simulink model "Q_estimation"  (R2021a)
settings: Solver=ode3  StartTime=0.0  StopTime=40  FixedStep=t_sim  RelTol=1e-3
values from neighbouring files (symbols this model uses):
  B0 = [0.1331 -0.0121 0.3981]    [Q_parameter.m]
  eul_0 = [0;0;0]    [Q_parameter.m]    (also in R_parameter.m)
  G0 = [0 0 9.81]    [Q_parameter.m]    (also in R_parameter.m = [0; 0; 9.81])
  k = 1    [Q_parameter.m]
  la = 9e-2    (= 0.09)    [Q_parameter.m]
  lc = 5e-2    (= 0.05)    [Q_parameter.m]
  ma = 9e-3    (= 0.009)    [Q_parameter.m]
  mc = 5e-3    (= 0.005)    [Q_parameter.m]
undefined symbols (not defined in the file or in its folder): DiscIntNeverNeededParam
libraries: sharedtransform x6, aerolibutil x4, sharedutil x3
settings Model: Creator=quangtruc  LastModifiedBy=quangtruc

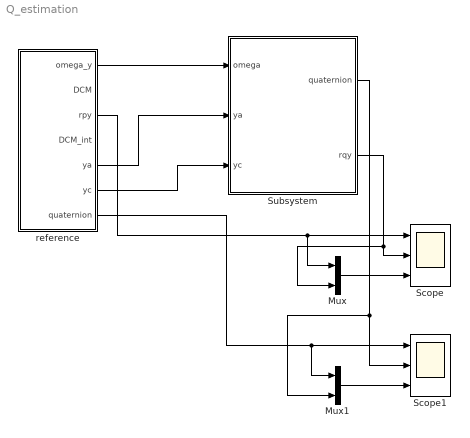
== system Q_estimation ==
  Mux : Mux  Inputs=2
  Mux1 : Mux  Inputs=2
  Scope : Scope  NumInputPorts=3
  Scope1 : Scope  NumInputPorts=3
  Subsystem : Subsystem
  reference : Subsystem
  wires:
  reference/1(omega_y) -> Subsystem/1(omega)
  reference/5(ya) -> Subsystem/2(ya)
  reference/6(yc) -> Subsystem/3(yc)
  Mux1/1 -> Scope1/3
  Mux/1 -> Scope/3
  Subsystem/2(rqy) -> Mux/2, Scope/2
  reference/3(rpy) -> Mux/1, Scope/1
  Subsystem/1(quaternion) -> Mux1/2, Scope1/2
  reference/7(quaternion) -> Scope1/1, Mux1/1

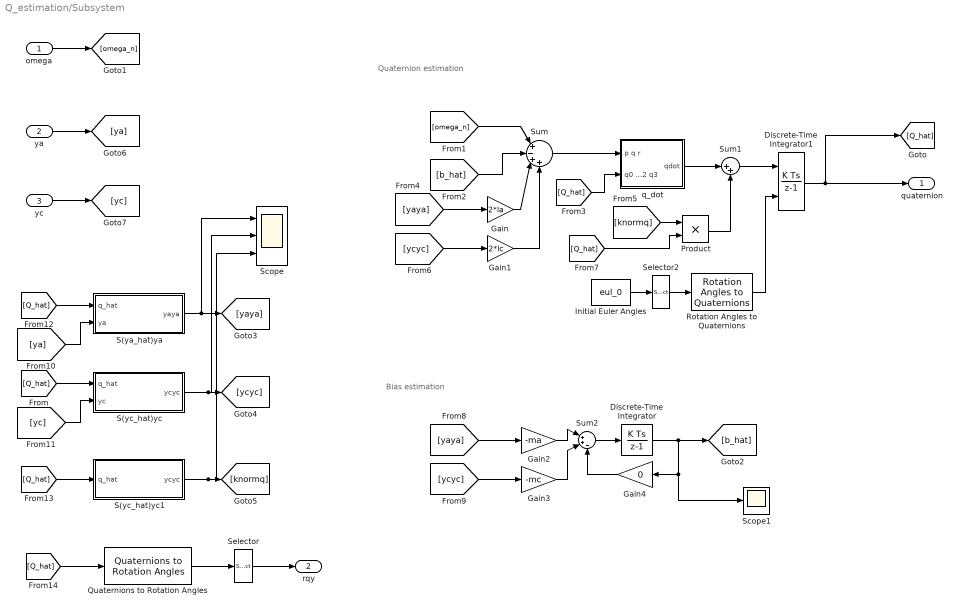
== system Q_estimation/Subsystem ==
  note: Bias estimation
  note: Quaternion estimation
  omega : Inport
  ya : Inport  Port=2
  yc : Inport  Port=3
  Discrete-Time Integrator : DiscreteIntegrator  SampleTime=-1  ICPrevOutput=DiscIntNeverNeededParam  ICPrevScaledInput=DiscIntNeverNeededParam
  Discrete-Time Integrator1 : DiscreteIntegrator  InitialConditionSource=external  SampleTime=-1  ICPrevOutput=DiscIntNeverNeededParam  ICPrevScaledInput=DiscIntNeverNeededParam
  Gain : Gain  Gain=2*la
  Gain1 : Gain  Gain=2*lc
  Gain2 : Gain  Gain=-ma
  Gain3 : Gain  Gain=-mc
  Gain4 : Gain  Gain=0
  Initial Euler Angles : Constant  Value=eul_0
  Product : Product
  Quaternions to Rotation Angles : sharedtransform/Quaternions to Rotation Angles  rotationOrder=ZYX  aMode=aMode
      settings: SourceProductBaseCode=AE,PW,DR,MT,UV,VE
  Rotation Angles to Quaternions : sharedtransform/Rotation Angles to Quaternions  rotationOrder=ZYX  aMode=aMode
      settings: SourceProductBaseCode=AE,PW,DR,MT,UV,VE
  S(ya_hat)ya : Subsystem
  S(yc_hat)yc : Subsystem
  S(yc_hat)yc1 : Subsystem
  Scope : Scope  NumInputPorts=3
  Scope1 : Scope
  Selector : Selector  InputPortWidth=3  IndexOptions=Index vector (dialog)  Indices=[3 2 1]  OutputSizes=1
  Selector2 : Selector  InputPortWidth=3  IndexOptions=Index vector (dialog)  Indices=[3 2 1]  OutputSizes=1
  Sum : Sum  Inputs=|+-++
  Sum1 : Sum  Inputs=|++
  Sum2 : Sum  Inputs=|++-
  q_dot : Subsystem
  quaternion : Outport  VectorParamsAs1DForOutWhenUnconnected=off
  rqy : Outport  Port=2  VectorParamsAs1DForOutWhenUnconnected=off
  wires:
  Initial Euler Angles/1 -> Selector2/1
  Rotation Angles to Quaternions/1 -> Discrete-Time Integrator1/2
  Discrete-Time Integrator1/1 -> [Q_hat], quaternion/1
  Selector2/1 -> Rotation Angles to Quaternions/1
  [omega_n] -> Sum/1
  Sum/1 -> q_dot/1(p q r)
  [b_hat] -> Sum/2
  Sum1/1 -> Discrete-Time Integrator1/1
  [Q_hat] -> q_dot/2(q0 q1 q2 q3)
  [yaya] -> Gain/1
  [ycyc] -> Gain1/1
  Gain/1 -> Sum/3
  Gain1/1 -> Sum/4
  [knormq] -> Product/1
  [Q_hat] -> Product/2
  [ycyc] -> Gain3/1
  [yaya] -> Gain2/1
  Gain2/1 -> Sum2/1
  Gain3/1 -> Sum2/2
  Sum2/1 -> Discrete-Time Integrator/1
  Discrete-Time Integrator/1 -> Gain4/1, Scope1/1, [b_hat]
  omega/1 -> [omega_n]
  ya/1 -> [ya]
  yc/1 -> [yc]
  [Q_hat] -> S(ya_hat)ya/1(q_hat)
  S(ya_hat)ya/1(yaya) -> Scope/1, [yaya]
  S(yc_hat)yc/1(ycyc) -> Scope/2, [ycyc]
  [Q_hat] -> S(yc_hat)yc/1(q_hat)
  [ya] -> S(ya_hat)ya/2(ya)
  [yc] -> S(yc_hat)yc/2(yc)
  S(yc_hat)yc1/1(ycyc) -> Scope/3, [knormq]
  [Q_hat] -> S(yc_hat)yc1/1(q_hat)
  Quaternions to Rotation Angles/1 -> Selector/1
  [Q_hat] -> Quaternions to Rotation Angles/1
  Selector/1 -> rqy/1
  Gain4/1 -> Sum2/3
  q_dot/1(qdot) -> Sum1/1
  Product/1 -> Sum1/2

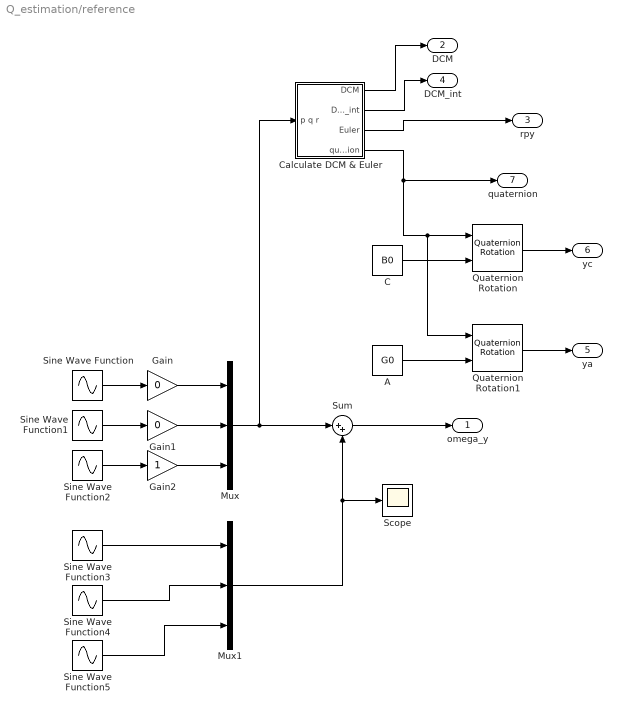
== system Q_estimation/reference ==
  A : Constant  Value=G0
  C : Constant  Value=B0
  "Calculate DCM & Euler " : Subsystem
  Gain : Gain  Gain=0
  Gain1 : Gain  Gain=0
  Gain2 : Gain
  Mux : Mux  Inputs=3
  Mux1 : Mux  Inputs=3
  Quaternion Rotation : aerolibutil/Quaternion Rotation
  Quaternion Rotation1 : aerolibutil/Quaternion Rotation
  Scope : Scope
  Sine Wave Function : Sin  SampleTime=0
  Sine Wave Function1 : Sin  SampleTime=0
  Sine Wave Function2 : Sin  Amplitude=0.5  Frequency=0.5  SampleTime=0
  Sine Wave Function3 : Sin  Amplitude=0.01  Frequency=0.1  SampleTime=0
  Sine Wave Function4 : Sin  Amplitude=0.015  Frequency=0.02  SampleTime=0
  Sine Wave Function5 : Sin  Amplitude=0.011  Frequency=0.005  SampleTime=0
  Sum : Sum  Inputs=|++
  omega_y : Outport
  DCM : Outport  Port=2
  rpy : Outport  Port=3
  DCM_int : Outport  Port=4
  ya : Outport  Port=5
  yc : Outport  Port=6
  quaternion : Outport  Port=7
  wires:
  "Calculate DCM & Euler "/1(DCM) -> DCM/1
  "Calculate DCM & Euler "/2(DCM_int) -> DCM_int/1
  "Calculate DCM & Euler "/3(Euler) -> rpy/1
  Gain/1 -> Mux/1
  Sine Wave Function/1 -> Gain/1
  Sine Wave Function1/1 -> Gain1/1
  Sine Wave Function2/1 -> Gain2/1
  Gain1/1 -> Mux/2
  Gain2/1 -> Mux/3
  Mux/1 -> "Calculate DCM & Euler "/1("p q r "), Sum/1
  Mux1/1 -> Scope/1, Sum/2
  Sum/1 -> omega_y/1
  "Calculate DCM & Euler "/4(quaternion) -> quaternion/1, Quaternion Rotation1/1, Quaternion Rotation/1
  C/1 -> Quaternion Rotation/2
  Quaternion Rotation/1 -> yc/1
  A/1 -> Quaternion Rotation1/2
  Quaternion Rotation1/1 -> ya/1
  Sine Wave Function3/1 -> Mux1/1
  Sine Wave Function4/1 -> Mux1/2
  Sine Wave Function5/1 -> Mux1/3

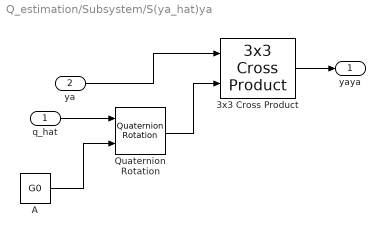
== system Q_estimation/Subsystem/S(ya_hat)ya ==
  q_hat : Inport
  ya : Inport  Port=2
  3x3 Cross Product : sharedutil/3x3 Cross Product  aMode=aMode
      settings: SourceProductBaseCode=AE,PW,DR,MT,UV,VE
  A : Constant  Value=G0
  Quaternion Rotation : aerolibutil/Quaternion Rotation
  yaya : Outport
  wires:
  q_hat/1 -> Quaternion Rotation/1
  A/1 -> Quaternion Rotation/2
  3x3 Cross Product/1 -> yaya/1
  ya/1 -> 3x3 Cross Product/1
  Quaternion Rotation/1 -> 3x3 Cross Product/2

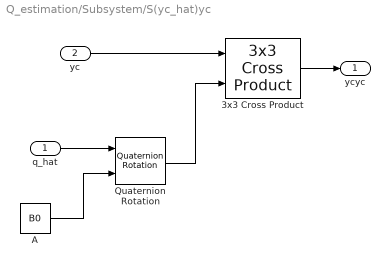
== system Q_estimation/Subsystem/S(yc_hat)yc ==
  q_hat : Inport
  yc : Inport  Port=2
  3x3 Cross Product : sharedutil/3x3 Cross Product  aMode=aMode
      settings: SourceProductBaseCode=AE,PW,DR,MT,UV,VE
  A : Constant  Value=B0
  Quaternion Rotation : aerolibutil/Quaternion Rotation
  ycyc : Outport
  wires:
  q_hat/1 -> Quaternion Rotation/1
  A/1 -> Quaternion Rotation/2
  3x3 Cross Product/1 -> ycyc/1
  yc/1 -> 3x3 Cross Product/1
  Quaternion Rotation/1 -> 3x3 Cross Product/2

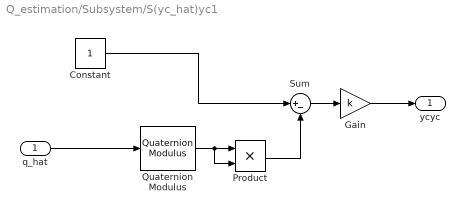
== system Q_estimation/Subsystem/S(yc_hat)yc1 ==
  q_hat : Inport
  Constant : Constant
  Gain : Gain  Gain=k
  Product : Product
  Quaternion Modulus : sharedutil/Quaternion Modulus  aMode=aMode
      settings: SourceProductBaseCode=AE,PW,DR,MT,UV,VE
  Sum : Sum  Inputs=|+-
  ycyc : Outport
  wires:
  Gain/1 -> ycyc/1
  q_hat/1 -> Quaternion Modulus/1
  Quaternion Modulus/1 -> Product/2, Product/1
  Product/1 -> Sum/2
  Sum/1 -> Gain/1
  Constant/1 -> Sum/1

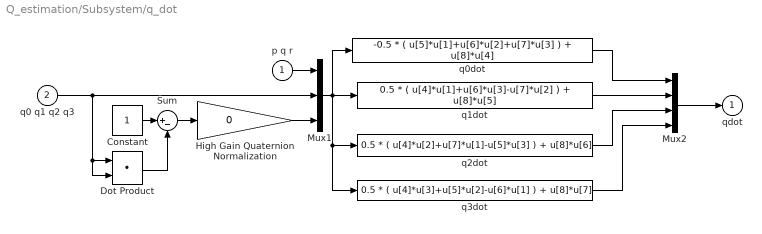
== system Q_estimation/Subsystem/q_dot ==
  p q r : Inport
  q0 q1 q2 q3 : Inport  Port=2
  Constant : Constant
  Dot Product : DotProduct  OutDataTypeStr=Inherit: Inherit via internal rule
  High Gain Quaternion Normalization : Gain  Gain=0  SaturateOnIntegerOverflow=on  OutDataTypeStr=Inherit: Same as input  ParamDataTypeStr=Inherit: Same as input
  Mux1 : Mux  Inputs=[3 4 1]
  Mux2 : Mux
  Sum : Sum  Inputs=|+-  InputSameDT=on  SaturateOnIntegerOverflow=on  OutDataTypeStr=Inherit: Same as first input
  q0dot : Fcn  Expr=-0.5 * ( u[5]*u[1]+u[6]*u[2]+u[7]*u[3] ) + u[8]*u[4]
  q1dot : Fcn  Expr=0.5 * ( u[4]*u[1]+u[6]*u[3]-u[7]*u[2] ) + u[8]*u[5]
  q2dot : Fcn  Expr=0.5 * ( u[4]*u[2]+u[7]*u[1]-u[5]*u[3] ) + u[8]*u[6]
  q3dot : Fcn  Expr=0.5 * ( u[4]*u[3]+u[5]*u[2]-u[6]*u[1] ) + u[8]*u[7]
  qdot : Outport  InitialOutput=0  VectorParamsAs1DForOutWhenUnconnected=off
  wires:
  q0 q1 q2 q3/1 -> Dot Product/1, Dot Product/2, Mux1/2
  q0dot/1 -> Mux2/1
  Constant/1 -> Sum/1
  Mux1/1 -> q2dot/1, q3dot/1, q0dot/1, q1dot/1
  Mux2/1 -> qdot/1
  q2dot/1 -> Mux2/3
  p q r/1 -> Mux1/1
  High Gain Quaternion Normalization/1 -> Mux1/3
  Dot Product/1 -> Sum/2
  q3dot/1 -> Mux2/4
  Sum/1 -> High Gain Quaternion Normalization/1
  q1dot/1 -> Mux2/2

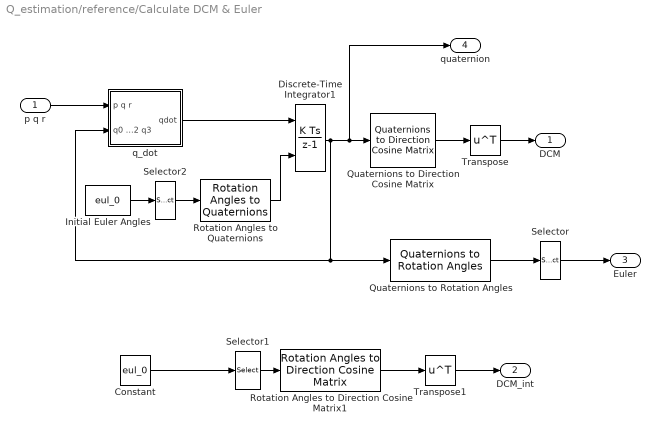
== system Q_estimation/reference/Calculate DCM & Euler  ==
  "p q r " : Inport
  Constant : Constant  Value=eul_0
  Discrete-Time Integrator1 : DiscreteIntegrator  InitialConditionSource=external  SampleTime=-1  ICPrevOutput=DiscIntNeverNeededParam  ICPrevScaledInput=DiscIntNeverNeededParam
  Initial Euler Angles : Constant  Value=eul_0
  Quaternions to Direction Cosine Matrix : sharedtransform/Quaternions to  Direction Cosine Matrix  aMode=aMode
      settings: SourceProductBaseCode=AE,PW,DR,MT,UV,VE
  Quaternions to Rotation Angles : sharedtransform/Quaternions to Rotation Angles  rotationOrder=ZYX  aMode=aMode
      settings: SourceProductBaseCode=AE,PW,DR,MT,UV,VE
  Rotation Angles to Direction Cosine Matrix1 : sharedtransform/Rotation Angles to Direction Cosine Matrix  rotationOrder=ZYX  aMode=aMode
      settings: SourceProductBaseCode=AE,PW,DR,MT,UV,VE
  Rotation Angles to Quaternions : sharedtransform/Rotation Angles to Quaternions  rotationOrder=ZYX  aMode=aMode
      settings: SourceProductBaseCode=AE,PW,DR,MT,UV,VE
  Selector : Selector  InputPortWidth=3  IndexOptions=Index vector (dialog)  Indices=[3 2 1]  OutputSizes=1
  Selector1 : Selector  InputPortWidth=3  IndexOptions=Index vector (dialog)  Indices=[3 2 1]  OutputSizes=1
  Selector2 : Selector  InputPortWidth=3  IndexOptions=Index vector (dialog)  Indices=[3 2 1]  OutputSizes=1
  Transpose : Math  Operator=transpose  SignedPower=on  SaturateOnIntegerOverflow=on
  Transpose1 : Math  Operator=transpose  SignedPower=on  SaturateOnIntegerOverflow=on
  q_dot : Subsystem
  DCM : Outport  VectorParamsAs1DForOutWhenUnconnected=off
  DCM_int : Outport  Port=2  VectorParamsAs1DForOutWhenUnconnected=off
  Euler : Outport  Port=3  VectorParamsAs1DForOutWhenUnconnected=off
  quaternion : Outport  Port=4  VectorParamsAs1DForOutWhenUnconnected=off
  wires:
  Rotation Angles to Direction Cosine Matrix1/1 -> Transpose1/1
  Transpose1/1 -> DCM_int/1
  Selector1/1 -> Rotation Angles to Direction Cosine Matrix1/1
  Constant/1 -> Selector1/1
  Quaternions to Rotation Angles/1 -> Selector/1
  "p q r "/1 -> q_dot/1(p q r)
  Initial Euler Angles/1 -> Selector2/1
  q_dot/1(qdot) -> Discrete-Time Integrator1/1
  Rotation Angles to Quaternions/1 -> Discrete-Time Integrator1/2
  Selector2/1 -> Rotation Angles to Quaternions/1
  Discrete-Time Integrator1/1 -> quaternion/1, Quaternions to Direction Cosine Matrix/1, q_dot/2(q0 q1 q2 q3), Quaternions to Rotation Angles/1
  Quaternions to Direction Cosine Matrix/1 -> Transpose/1
  Transpose/1 -> DCM/1
  Selector/1 -> Euler/1

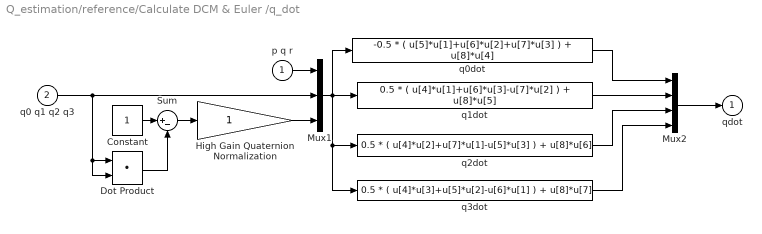
== system Q_estimation/reference/Calculate DCM & Euler /q_dot ==
  p q r : Inport
  q0 q1 q2 q3 : Inport  Port=2
  Constant : Constant
  Dot Product : DotProduct  OutDataTypeStr=Inherit: Inherit via internal rule
  High Gain Quaternion Normalization : Gain  SaturateOnIntegerOverflow=on  OutDataTypeStr=Inherit: Same as input  ParamDataTypeStr=Inherit: Same as input
  Mux1 : Mux  Inputs=[3 4 1]
  Mux2 : Mux
  Sum : Sum  Inputs=|+-  InputSameDT=on  SaturateOnIntegerOverflow=on  OutDataTypeStr=Inherit: Same as first input
  q0dot : Fcn  Expr=-0.5 * ( u[5]*u[1]+u[6]*u[2]+u[7]*u[3] ) + u[8]*u[4]
  q1dot : Fcn  Expr=0.5 * ( u[4]*u[1]+u[6]*u[3]-u[7]*u[2] ) + u[8]*u[5]
  q2dot : Fcn  Expr=0.5 * ( u[4]*u[2]+u[7]*u[1]-u[5]*u[3] ) + u[8]*u[6]
  q3dot : Fcn  Expr=0.5 * ( u[4]*u[3]+u[5]*u[2]-u[6]*u[1] ) + u[8]*u[7]
  qdot : Outport  InitialOutput=0  VectorParamsAs1DForOutWhenUnconnected=off
  wires:
  q0 q1 q2 q3/1 -> Dot Product/1, Dot Product/2, Mux1/2
  q0dot/1 -> Mux2/1
  Constant/1 -> Sum/1
  Mux1/1 -> q2dot/1, q3dot/1, q0dot/1, q1dot/1
  Mux2/1 -> qdot/1
  q2dot/1 -> Mux2/3
  p q r/1 -> Mux1/1
  High Gain Quaternion Normalization/1 -> Mux1/3
  Dot Product/1 -> Sum/2
  q3dot/1 -> Mux2/4
  Sum/1 -> High Gain Quaternion Normalization/1
  q1dot/1 -> Mux2/2
